simulink library "aerolibatmos"  (Simulink 5.0)
values from neighbouring files (symbols this model uses):
  s = aeroliblist    [asbhelp.m]
undefined symbols (not defined in the file or in its folder): kg, m
libraries: aerolibconvert x5
settings Model: ForwardingTableString=||__slOldName__||aerolibatmos/COESA Atmosphere Model||__slNewName__||aerolibprivatev1p5/COESA Atmosphere Model||__slOldName__||aerolibatmos/ISA Atmosphere Model||__slNewName__||aerolibatmos2/ISA Atmosphere Model  Creator=sgage  LastModifiedBy=sgage  ExtModeAutoUpdateStatusClock=off  TargetHWChar=2  TargetHWWordLengths=8,16,32,32

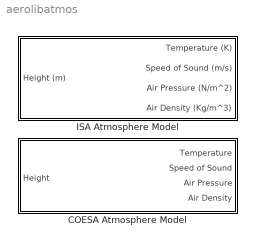
== system aerolibatmos ==
  COESA Atmosphere Model : Subsystem  mask(COESA Atmosphere Model){units=Metric}
      mask help:
      | Calculate 1976 COESA-extended U.S. Standard Atmosphere. Given geopotential altitude, calculate absolute temperature, pressure, and density using standard interpolation formulas (linear in temperature and logarithmic in pressure).
      |
      | Extrapolate temperature linearly and pressure  logarithmically beyond the range
      |            0 <= altitude <= 84852 m
      |
      | Density is calculated using a perfect gas relationship.
      |
      | Data used is from the 15-OCT-1976 COESA extensions to the U.S. Standard Atmosphere, 1976, published by the U.S. Government Printing Office, Washington, D.C.
      |
      | The unit system selected applies to both input and outputs.
      mask init:
      | [ports] = aeroicon('aeroblkcoesa','icon');
      mask Help: web(asbhelp);
      mask StyleString: popup(Metric|English)
      mask Display:
      | port_label(ports(1).type,ports(1).port,ports(1).txt);
      | port_label(ports(2).type,ports(2).port,ports(2).txt);
      | port_label(ports(3).type,ports(3).port,ports(3).txt);
      | port_label(ports(4).type,ports(4).port,ports(4).txt);
      | port_label(ports(5).type,ports(5).port,ports(5).txt);
  ISA Atmosphere Model : Subsystem  mask(International Standard Atmosphere Model){}
      mask help: Compute International Standard Atmosphere (ISA) model for altitudes between 0 Km and 20 Km.
      mask init:
      | g=9.80665; % m/s
      | gamma = 1.4;
      | R = 287.0531; %J/Kg/K
      | L = 0.0065; % K/m
      | h_trop = 11000; % m
      | rho0 = 1.225; %Kg/m^3
      | P0 = 101325; % Pa
      | T0 = 288.15; % K
      mask Help: web(asbhelp('isaatmospheremodel'));

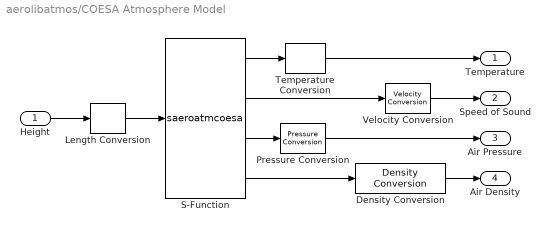
== system aerolibatmos/COESA Atmosphere Model ==
  Height : Inport
  Density Conversion : aerolibconvert/Density Conversion  IU=kg/m^3  OU=kg/m^3
  Length Conversion : aerolibconvert/Length Conversion  IU=m  OU=m
  Pressure Conversion : aerolibconvert/Pressure Conversion  IU=Pa  OU=Pa
  S-Function : S-Function  FunctionName=saeroatmcoesa  SFunctionModules=aeroatmcoesa
  Temperature Conversion : aerolibconvert/Temperature Conversion  IU=K  OU=K
  Velocity Conversion : aerolibconvert/Velocity Conversion  IU=m/s  OU=m/s
  Temperature : Outport
  Speed of Sound : Outport  Port=2
  Air Pressure : Outport  Port=3
  Air Density : Outport  Port=4
  wires:
  Density Conversion/1 -> Air Density/1
  Pressure Conversion/1 -> Air Pressure/1
  Height/1 -> Length Conversion/1
  Temperature Conversion/1 -> Temperature/1
  S-Function/4 -> Density Conversion/1
  S-Function/3 -> Pressure Conversion/1
  S-Function/1 -> Temperature Conversion/1
  S-Function/2 -> Velocity Conversion/1
  Velocity Conversion/1 -> Speed of Sound/1
  Length Conversion/1 -> S-Function/1

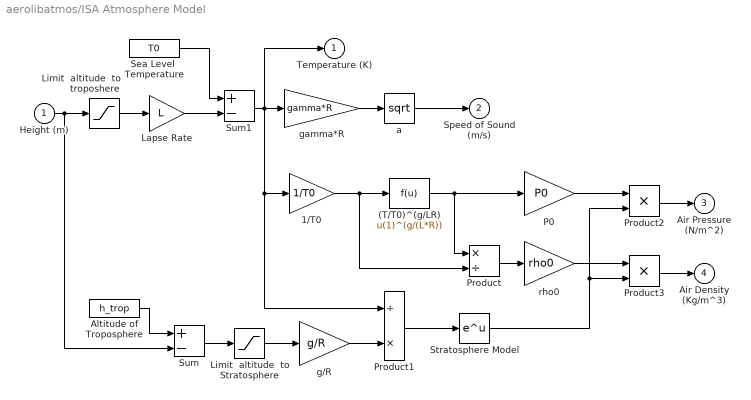
== system aerolibatmos/ISA Atmosphere Model ==
  Height (m) : Inport
  (T/T0)^(g/LR) : Fcn  Expr=u(1)^(g/(L*R))
  1/T0 : Gain  Gain=1/T0  SaturateOnIntegerOverflow=on
  Altitude of Troposphere : Constant  Value=h_trop
  Lapse Rate : Gain  Gain=L  SaturateOnIntegerOverflow=on
  Limit  altitude  to Stratosphere : Saturate  UpperLimit=0  LowerLimit=h_trop-20000
  Limit  altitude  to troposhere : Saturate  UpperLimit=h_trop  LowerLimit=0
  P0 : Gain  Gain=P0  SaturateOnIntegerOverflow=on
  Product : Product  Inputs=*/  SaturateOnIntegerOverflow=on  InputSameDT=on
  Product1 : Product  Inputs=/*  SaturateOnIntegerOverflow=on  InputSameDT=on
  Product2 : Product  SaturateOnIntegerOverflow=on  InputSameDT=on
  Product3 : Product  SaturateOnIntegerOverflow=on  InputSameDT=on
  Sea Level  Temperature : Constant  Value=T0
  Stratosphere Model : Math
  Sum : Sum  Inputs=+-  SaturateOnIntegerOverflow=on  InputSameDT=on
  Sum1 : Sum  Inputs=+-  SaturateOnIntegerOverflow=on  InputSameDT=on
  a : Math  Operator=sqrt
  g/R : Gain  Gain=g/R  SaturateOnIntegerOverflow=on
  gamma*R : Gain  Gain=gamma*R  SaturateOnIntegerOverflow=on
  rho0 : Gain  Gain=rho0  SaturateOnIntegerOverflow=on
  Temperature (K) : Outport  InitialOutput=0
  "Speed of Sound (m/s) " : Outport  Port=2  InitialOutput=0
  "Air Pressure (N/m^2) " : Outport  Port=3  InitialOutput=0
  Air Density (Kg/m^3) : Outport  Port=4  InitialOutput=0
  wires:
  Limit  altitude  to Stratosphere/1 -> g/R/1
  Sum/1 -> Limit  altitude  to Stratosphere/1
  Altitude of Troposphere/1 -> Sum/1
  Product1/1 -> Stratosphere Model/1
  g/R/1 -> Product1/2
  Stratosphere Model/1 -> Product3/2, Product2/2
  Product3/1 -> Air Density (Kg/m^3)/1
  rho0/1 -> Product3/1
  Product2/1 -> "Air Pressure (N/m^2) "/1
  P0/1 -> Product2/1
  Sea Level  Temperature/1 -> Sum1/1
  Lapse Rate/1 -> Sum1/2
  Sum1/1 -> Product1/1, 1/T0/1, gamma*R/1, Temperature (K)/1
  a/1 -> "Speed of Sound (m/s) "/1
  gamma*R/1 -> a/1
  1/T0/1 -> (T/T0)^(g/LR)/1, Product/2
  (T/T0)^(g/LR)/1 -> P0/1, Product/1
  Product/1 -> rho0/1
  Limit  altitude  to troposhere/1 -> Lapse Rate/1
  Height (m)/1 -> Sum/2, Limit  altitude  to troposhere/1
